simulink model "Helicoper_3DOF"  (R2019b)
settings: Solver=VariableStepAuto  StartTime=0.0  StopTime=10.0  RelTol=1e-3
values from neighbouring files (symbols this model uses):
  A = double((subs(A_mat)))    [Linearize.m]    (also in Linearize_old.m)
  B = double((subs(B_mat)))    [Linearize.m]    (also in Linearize_old.m)
  D = zeros(size(3,2))    [Linearize.m]    (also in Linearize_old.m)
settings Model: Creator=boateng  LastModifiedBy=boateng

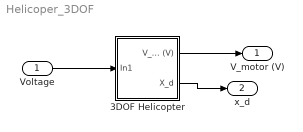
== system Helicoper_3DOF ==
  Voltage : Inport
  3DOF Helicopter : Subsystem
      mask Display:
      | pic = imread("IST_quanser_Heli.png")
      | 
      | set_param(gcb, 'UserDataPersistent', 'on');
      | 
      | ud.pic = pic
      | 
      | set_param(gcb, 'UserData', ud)
      | 
      | ud = get_param(gcb, 'UserData')
      | 
      | image(ud.pic)
  V_motor (V) : Outport
  x_d : Outport  Port=2
  wires:
  Voltage/1 -> 3DOF Helicopter/1(In1)
  3DOF Helicopter/1(V_motor (V)) -> V_motor (V)/1
  3DOF Helicopter/2(X_d) -> x_d/1

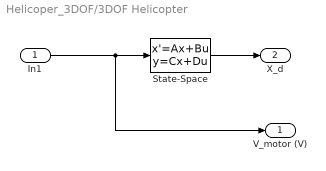
== system Helicoper_3DOF/3DOF Helicopter ==
  In1 : Inport
  State-Space : StateSpace  A=A  B=B  C=D  D=zeros(6,2)  InitialCondition=0
  V_motor (V) : Outport
  X_d : Outport  Port=2
  wires:
  State-Space/1 -> X_d/1
  In1/1 -> V_motor (V)/1, State-Space/1
